simulink model "slexMonostaticRadarExample"  (R2015b)
settings: Solver=FixedStepDiscrete  StartTime=0.0  StopTime=99/paramRadar.prf  RelTol=1e-3
PreLoadFcn:
  | helperslexMonostaticRadarParam()
undefined symbols (not defined in the file or in its folder): paramRadar
libraries: phasedenvlib x4, phaseddetectlib x3, phasedtxrxlib x2, simulink x1, phasedwavlib x1, phasedmisclib x1
CloseFcn:
  | clear paramRadar
Description:
  | Monostatic Radar with One Target
settings Model: ModifiedByFormat=The MathWorks Inc.  Creator=The MathWorks, Inc.  LastModifiedBy=The MathWorks Inc.
settings DataIOCC: SaveFormat=Array  SaveOutput=off  SaveTime=off
settings OptimizationCC: ExpressionDepthLimit=2147483647
settings DebuggingCC: ReadBeforeWriteMsg=DisableAll  WriteAfterWriteMsg=DisableAll  WriteAfterReadMsg=DisableAll  UnderspecifiedInitializationDetection=Classic  MergeDetectMultiDrivingBlocksExec=none  SolverPrmCheckMsg=warning  MultiTaskDSMMsg=none  FcnCallInpInsideContextMsg=UseLocalSettings  StateNameClashWarn=warning
settings HardwareCC: ProdBitPerPointer=32  ProdLargestAtomicFloat=None  ProdIntDivRoundTo=Undefined  ProdEndianess=Unspecified  ProdWordSize=32  ProdHWDeviceType=32-bit Generic
settings ModelReferenceCC: UpdateModelReferenceTargets=IfOutOfDate
settings SFSimCC: SFSimEcho=off  SimParseCustomCode=off
settings GRTTargetCC: GeneratePreprocessorConditionals=Disable all  CombineOutputUpdateFcns=off  GRTInterface=on
settings ConfigComp: CovModelRefEnable=Off  CovSFcnEnable=off

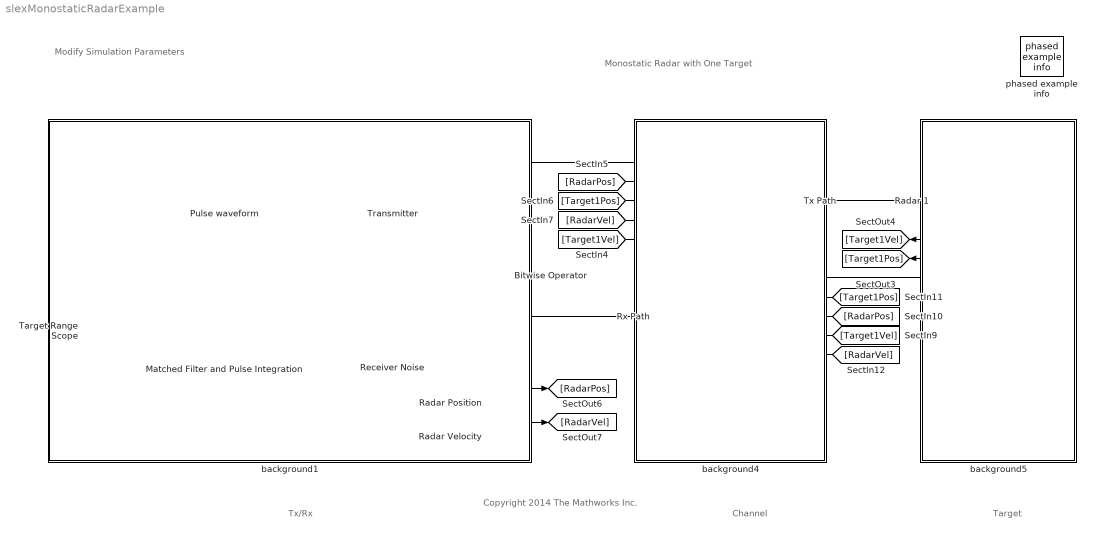
== system slexMonostaticRadarExample ==
  note: Monostatic Radar with One Target
  note: Tx/Rx
  note: Channel
  note: Target
  note: Modify Simulation Parameters
  note: Copyright 2014 The Mathworks Inc.
  Bitwise Operator : simulink/Logic and Bit Operations/Bitwise Operator  logicop=NOT  UseBitMask=off  BitMask=bin2dec('11011001')  BitMaskRealWorld=Stored Integer
  Matched Filter and Pulse Integration : Subsystem
      mask Display: disp('Signal Processing')
  Pulse waveform : phasedwavlib/Rectangular Waveform  SampleRate=paramRadar.fs  PulseWidth=1/paramRadar.pulseBw  PRF=paramRadar.prf  OutputFormat=Pulses  NumSamples=100  NumPulses=1  SimulateUsing=Interpreted execution
  Radar 1 : Subsystem
      mask Display:
      | disp('Target')
      | port_label('output',1,'Y');
      | port_label('output',2,'Pos');
      | port_label('output',3,'Vel');
  Radar Position : Constant  Value=[ 0; 0; 0 ]  SampleTime=1/paramRadar.prf
  Radar Velocity : Constant  Value=[ 0; 0; 0 ]  SampleTime=1/paramRadar.prf
  Receiver Noise : phasedtxrxlib/Receiver Preamp  Gain=20  LossFactor=0  NoiseMethod=Noise temperature  NoiseFigure=0  ReferenceTemperature=290  NoisePower=0  EnableInputPort=on  PhaseNoiseInputPort=off  SeedSource=Auto  Seed=0  SimulateUsing=Interpreted execution
  Rx Path : phasedenvlib/Free Space  PropagationSpeed=paramRadar.propSpeed  OperatingFrequency=paramRadar.fc  TwoWayPropagation=off  MaximumDistanceSource=Property  MaximumDistance=10e3  SimulateUsing=Interpreted execution
  Target Range Scope : ArrayPlot
  Transmitter : phasedtxrxlib/Transmitter  PeakPower=paramRadar.peakPower  Gain=paramRadar.txGain  LossFactor=0  InUseOutputPort=on  CoherentOnTransmit=on  PhaseNoiseOutputPort=off  SeedSource=Auto  Seed=0  SimulateUsing=Interpreted execution
  Tx Path : phasedenvlib/Free Space  PropagationSpeed=paramRadar.propSpeed  OperatingFrequency=paramRadar.fc  TwoWayPropagation=off  MaximumDistanceSource=Property  MaximumDistance=10e3  SimulateUsing=Interpreted execution
  background1 : Subsystem  Description=Jammer
      mask Display: disp('')
  background4 : Subsystem  Description=Jammer
      mask Display: disp('')
  background5 : Subsystem  Description=Jammer
      mask Display: disp('')
  phased example info : phasedmisclib/phased example info  SystemSampleTime=-1
  wires:
  Pulse waveform/1 -> Transmitter/1
  Receiver Noise/1 -> Matched Filter and Pulse Integration/1(In1)
  Matched Filter and Pulse Integration/1(Out1) -> Target Range Scope/1
  Transmitter/2 -> Bitwise Operator/1
  Bitwise Operator/1 -> Receiver Noise/2
  [RadarVel] -> Tx Path/4
  [Target1Pos] -> Tx Path/3
  [Target1Vel] -> Tx Path/5
  [RadarPos] -> Tx Path/2
  [Target1Vel] -> Rx Path/4
  [Target1Pos] -> Rx Path/2
  [RadarPos] -> Rx Path/3
  [RadarVel] -> Rx Path/5
  Radar 1/2(P) -> [Target1Pos]
  Tx Path/1 -> Radar 1/1(In1)
  Radar 1/1(Out1) -> Rx Path/1
  Transmitter/1 -> Tx Path/1
  Rx Path/1 -> Receiver Noise/1
  Radar Position/1 -> [RadarPos]
  Radar Velocity/1 -> [RadarVel]
  Radar 1/3(V) -> [Target1Vel]

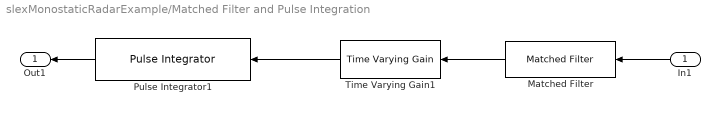
== system slexMonostaticRadarExample/Matched Filter and Pulse Integration ==
  In1 : Inport
  Matched Filter : phaseddetectlib/Matched Filter  CoefficientsSource=Property  Coefficients=paramRadar.matchingCoeff  SpectrumWindow=None  CustomSpectrumWindow=@hamming  SpectrumRange=[ 0, 1e5 ]  SidelobeAttenuation=30  Beta=0.5  Nbar=4  GainOutputPort=off  SimulateUsing=Interpreted execution
  Pulse Integrator1 : phaseddetectlib/Pulse Integrator  CoherentFlag=Noncoherent  N=10  V=0
  Time Varying Gain1 : phaseddetectlib/Time Varying Gain  RangeLoss=paramRadar.rangeLoss  ReferenceLoss=paramRadar.referenceLoss  SimulateUsing=Interpreted execution
  Out1 : Outport
  wires:
  In1/1 -> Matched Filter/1
  Time Varying Gain1/1 -> Pulse Integrator1/1
  Matched Filter/1 -> Time Varying Gain1/1
  Pulse Integrator1/1 -> Out1/1

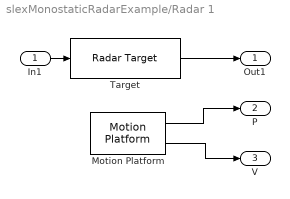
== system slexMonostaticRadarExample/Radar 1 ==
  In1 : Inport
  Motion Platform : phasedenvlib/Motion Platform  MotionModel=Velocity  InitialPosition=paramRadar.target1Pos  InitialVelocity=[ 0; 0; 0 ]  VelocitySource=Property  Velocity=paramRadar.target1Vel  AccelerationSource=Property  Acceleration=[0;0;0]  InitialOrientationAxes=eye( 3 )  OrientationAxesOutputPort=off  SimulateUsing=Interpreted execution
  Target : phasedenvlib/Radar Target  EnablePolarization=off  Mode=Monostatic  MeanRCSSource=Property  ScatteringMatrixSource=Property  MeanRCS=paramRadar.target1Rcs  ScatteringMatrix=eye( 2 )  Model=Nonfluctuating  PropagationSpeed=paramRadar.propSpeed  OperatingFrequency=paramRadar.fc  SeedSource=Auto  Seed=0  SimulateUsing=Interpreted execution
  Out1 : Outport
  P : Outport  Port=2
  V : Outport  Port=3
  wires:
  In1/1 -> Target/1
  Target/1 -> Out1/1
  Motion Platform/1 -> P/1
  Motion Platform/2 -> V/1

== system slexMonostaticRadarExample/background1 ==

== system slexMonostaticRadarExample/background4 ==

== system slexMonostaticRadarExample/background5 ==
